simulink model "ALL_JP360_DBW_V6_5_1103"  (R2022a)
settings: Solver=FixedStepAuto  StartTime=0.0  StopTime=inf  FixedStep=0.01  RelTol=1e-3  EnableMultiTasking=on
model workspace (MAT data in the model file):
  g = 9.8
undefined symbols (not defined in the file or in its folder): canChannel, delta_v_p, IPM_Line_C0, IPM_Line_C1, IPM_Line_C2, IPM_Line_C3, M, M_p, MRR_ObjDistX, MRR_ObjDistY, MRR_ObjFusionCamID, MRR_ObjFusionSig, MRR_ObjID, MRR_ObjRelVelX, MRR_ObjRelVelY, MRR_ObjType, MRR_ObjUpdFlg, none, obj_vaild, untracktime, V, videoinput
libraries: canfdmsglib x230, canfdlib x76, slpidlib x24, simulink x18, dspstat3 x14, ctrlSharedLib x1, simulink_extras x1, imaqlib x1, realtime_pacer_lib x1, dspvision x1, visionsinks x1
(part 45 of 55)

== system ALL_JP360_DBW_V6_5_1103/MsgFromCAN/VR_ADCU_MsgFromCAN/VR_ADCU_IPM_Traffic_01_0x670 ==
  VR_ADCU_IPM_Traffic_01_0x670FromInData : Inport  OutDataTypeStr=Bus:CAN_FD_MESSAGE_BUS
  Bus Creator : BusCreator  Inputs=11  OutDataTypeStr=Bus:VR_ADCU_IPM_Traffic_01_0x670  NonVirtualBus=on
  CAN FD Unpack : canfdmsglib/CAN FD Unpack  CANdbFile=HiFire_T360_P789_1R1V_Pri_Matrix_CAN_V2.3_20220810.dbc  MsgList=(none)  MsgName=IPM_Traffic_01_0x670  ProtocolMode=CAN FD  MsgIDType=Standard (11-bit identifier)  MsgIdentifier=1648  MsgLength=20  SignalInfo={'IPM_TrafficSign01_BlockCounter','13','11','BE','unsigned','Standard','0','1','0','0','2047';'IPM_TrafficSign01_Checksum','152','16','BE','unsigned','Standard','0','1','0','0','65535';'IPM_TrafficSign01_Confidence','86','6','BE','unsigned','Standard','0','2','0','0','100';'IPM_TrafficSign01_Count','56','8','BE','unsigned','Standard','0','1','0','0','255';'IPM_TrafficSign01_ID','21','8','BE','unsigned','Standard','0','1','0','0','255';'IPM_TrafficSign01_MsgCounter','136','4','BE','unsigned','Standard','0','1','0','0','15';'IPM_TrafficSign01_PositionX','25','12','BE','unsigned','Standard','0','0.0625','0','0','254.9375';'IPM_TrafficSign01_PositionY','43','14','BE','unsigned','Standard','0','0.0078125','-64','-64','63.9922';'IPM_TrafficSign01_PositionZ','49','10','BE','unsigned','Standard','0','0.05','0','0','51.15';'IPM_TrafficSign01_Shape','76','4','BE','unsigned','Standard','0','1','0','0','15';'IPM_TrafficSign01_Type','64','8','BE','unsigned','Standard','0','1','0','0','255'}  IDPort=off  TimestampPort=off  ErrorPort=off  RemotePort=off  LengthPort=off  StatusPort=off  BRSPort=off  ESIPort=off  DLCPort=off  ApplyMinMax=off
      settings: SourceProductBaseCode=ME,XP,VN  DataFormat=CANdb specified signals
  Data Type Conversion1 : DataTypeConversion  OutDataTypeStr=int16  SaturateOnIntegerOverflow=off  RndMeth=Floor
  Data Type Conversion10 : DataTypeConversion  OutDataTypeStr=int8  SaturateOnIntegerOverflow=off  RndMeth=Floor
  Data Type Conversion11 : DataTypeConversion  OutDataTypeStr=uint8  SaturateOnIntegerOverflow=off  RndMeth=Floor
  Data Type Conversion2 : DataTypeConversion  OutDataTypeStr=uint16  SaturateOnIntegerOverflow=off  RndMeth=Floor
  Data Type Conversion3 : DataTypeConversion  OutDataTypeStr=int8  SaturateOnIntegerOverflow=off  RndMeth=Floor
  Data Type Conversion4 : DataTypeConversion  OutDataTypeStr=uint8  SaturateOnIntegerOverflow=off  RndMeth=Floor
  Data Type Conversion5 : DataTypeConversion  OutDataTypeStr=uint8  SaturateOnIntegerOverflow=off  RndMeth=Floor
  Data Type Conversion6 : DataTypeConversion  OutDataTypeStr=int8  SaturateOnIntegerOverflow=off  RndMeth=Floor
  Data Type Conversion7 : DataTypeConversion  OutDataTypeStr=single  SaturateOnIntegerOverflow=off  RndMeth=Floor
  Data Type Conversion8 : DataTypeConversion  OutDataTypeStr=single  SaturateOnIntegerOverflow=off  RndMeth=Floor
  Data Type Conversion9 : DataTypeConversion  OutDataTypeStr=single  SaturateOnIntegerOverflow=off  RndMeth=Floor
  VR_ADCU_IPM_Traffic_01_0x670FromOutData : Outport  OutDataTypeStr=Bus:VR_ADCU_IPM_Traffic_01_0x670
  wires:
  CAN FD Unpack/1 -> Data Type Conversion1/1
  CAN FD Unpack/2 -> Data Type Conversion2/1
  CAN FD Unpack/3 -> Data Type Conversion3/1
  CAN FD Unpack/4 -> Data Type Conversion4/1
  CAN FD Unpack/5 -> Data Type Conversion5/1
  CAN FD Unpack/6 -> Data Type Conversion6/1
  CAN FD Unpack/7 -> Data Type Conversion7/1
  CAN FD Unpack/8 -> Data Type Conversion8/1
  CAN FD Unpack/9 -> Data Type Conversion9/1
  CAN FD Unpack/10 -> Data Type Conversion10/1
  CAN FD Unpack/11 -> Data Type Conversion11/1
  Data Type Conversion1/1 -> Bus Creator/1  "IPM_TrafficSign01_BlockCounter"
  Data Type Conversion2/1 -> Bus Creator/2  "IPM_TrafficSign01_Checksum"
  Data Type Conversion3/1 -> Bus Creator/3  "IPM_TrafficSign01_Confidence"
  Data Type Conversion4/1 -> Bus Creator/4  "IPM_TrafficSign01_Count"
  Data Type Conversion5/1 -> Bus Creator/5  "IPM_TrafficSign01_ID"
  Data Type Conversion6/1 -> Bus Creator/6  "IPM_TrafficSign01_MsgCounter"
  Data Type Conversion7/1 -> Bus Creator/7  "IPM_TrafficSign01_PositionX"
  Data Type Conversion8/1 -> Bus Creator/8  "IPM_TrafficSign01_PositionY"
  Data Type Conversion9/1 -> Bus Creator/9  "IPM_TrafficSign01_PositionZ"
  Data Type Conversion10/1 -> Bus Creator/10  "IPM_TrafficSign01_Shape"
  Data Type Conversion11/1 -> Bus Creator/11  "IPM_TrafficSign01_Type"
  Bus Creator/1 -> VR_ADCU_IPM_Traffic_01_0x670FromOutData/1  "VR_ADCU_IPM_Traffic_01_0x670FromOutData"
  VR_ADCU_IPM_Traffic_01_0x670FromInData/1 -> CAN FD Unpack/1  "VR_ADCU_IPM_Traffic_01_0x670FromInData"

== system ALL_JP360_DBW_V6_5_1103/MsgFromCAN/VR_ADCU_MsgFromCAN/VR_ADCU_IPM_Traffic_02_0x671 ==
  VR_ADCU_IPM_Traffic_02_0x671FromInData : Inport  OutDataTypeStr=Bus:CAN_FD_MESSAGE_BUS
  Bus Creator : BusCreator  Inputs=11  OutDataTypeStr=Bus:VR_ADCU_IPM_Traffic_02_0x671  NonVirtualBus=on
  CAN FD Unpack : canfdmsglib/CAN FD Unpack  CANdbFile=HiFire_T360_P789_1R1V_Pri_Matrix_CAN_V2.3_20220810.dbc  MsgList=(none)  MsgName=IPM_Traffic_02_0x671  ProtocolMode=CAN FD  MsgIDType=Standard (11-bit identifier)  MsgIdentifier=1649  MsgLength=20  SignalInfo={'IPM_TrafficSign02_BlockCounter','13','11','BE','unsigned','Standard','0','1','0','0','2047';'IPM_TrafficSign02_Checksum','152','16','BE','unsigned','Standard','0','1','0','0','65535';'IPM_TrafficSign02_Confidence','86','6','BE','unsigned','Standard','0','2','0','0','100';'IPM_TrafficSign02_Count','56','8','BE','unsigned','Standard','0','1','0','0','255';'IPM_TrafficSign02_ID','21','8','BE','unsigned','Standard','0','1','0','0','255';'IPM_TrafficSign02_MsgCounter','136','4','BE','unsigned','Standard','0','1','0','0','15';'IPM_TrafficSign02_PositionX','25','12','BE','unsigned','Standard','0','0.0625','0','0','254.9375';'IPM_TrafficSign02_PositionY','43','14','BE','unsigned','Standard','0','0.0078125','-64','-64','63.9922';'IPM_TrafficSign02_PositionZ','49','10','BE','unsigned','Standard','0','0.05','0','0','51.15';'IPM_TrafficSign02_Shape','76','4','BE','unsigned','Standard','0','1','0','0','15';'IPM_TrafficSign02_Type','64','8','BE','unsigned','Standard','0','1','0','0','255'}  IDPort=off  TimestampPort=off  ErrorPort=off  RemotePort=off  LengthPort=off  StatusPort=off  BRSPort=off  ESIPort=off  DLCPort=off  ApplyMinMax=off
      settings: SourceProductBaseCode=ME,XP,VN  DataFormat=CANdb specified signals
  Data Type Conversion1 : DataTypeConversion  OutDataTypeStr=int16  SaturateOnIntegerOverflow=off  RndMeth=Floor
  Data Type Conversion10 : DataTypeConversion  OutDataTypeStr=int8  SaturateOnIntegerOverflow=off  RndMeth=Floor
  Data Type Conversion11 : DataTypeConversion  OutDataTypeStr=uint8  SaturateOnIntegerOverflow=off  RndMeth=Floor
  Data Type Conversion2 : DataTypeConversion  OutDataTypeStr=uint16  SaturateOnIntegerOverflow=off  RndMeth=Floor
  Data Type Conversion3 : DataTypeConversion  OutDataTypeStr=int8  SaturateOnIntegerOverflow=off  RndMeth=Floor
  Data Type Conversion4 : DataTypeConversion  OutDataTypeStr=uint8  SaturateOnIntegerOverflow=off  RndMeth=Floor
  Data Type Conversion5 : DataTypeConversion  OutDataTypeStr=uint8  SaturateOnIntegerOverflow=off  RndMeth=Floor
  Data Type Conversion6 : DataTypeConversion  OutDataTypeStr=int8  SaturateOnIntegerOverflow=off  RndMeth=Floor
  Data Type Conversion7 : DataTypeConversion  OutDataTypeStr=single  SaturateOnIntegerOverflow=off  RndMeth=Floor
  Data Type Conversion8 : DataTypeConversion  OutDataTypeStr=single  SaturateOnIntegerOverflow=off  RndMeth=Floor
  Data Type Conversion9 : DataTypeConversion  OutDataTypeStr=single  SaturateOnIntegerOverflow=off  RndMeth=Floor
  VR_ADCU_IPM_Traffic_02_0x671FromOutData : Outport  OutDataTypeStr=Bus:VR_ADCU_IPM_Traffic_02_0x671
  wires:
  CAN FD Unpack/1 -> Data Type Conversion1/1
  CAN FD Unpack/2 -> Data Type Conversion2/1
  CAN FD Unpack/3 -> Data Type Conversion3/1
  CAN FD Unpack/4 -> Data Type Conversion4/1
  CAN FD Unpack/5 -> Data Type Conversion5/1
  CAN FD Unpack/6 -> Data Type Conversion6/1
  CAN FD Unpack/7 -> Data Type Conversion7/1
  CAN FD Unpack/8 -> Data Type Conversion8/1
  CAN FD Unpack/9 -> Data Type Conversion9/1
  CAN FD Unpack/10 -> Data Type Conversion10/1
  CAN FD Unpack/11 -> Data Type Conversion11/1
  Data Type Conversion1/1 -> Bus Creator/1  "IPM_TrafficSign02_BlockCounter"
  Data Type Conversion2/1 -> Bus Creator/2  "IPM_TrafficSign02_Checksum"
  Data Type Conversion3/1 -> Bus Creator/3  "IPM_TrafficSign02_Confidence"
  Data Type Conversion4/1 -> Bus Creator/4  "IPM_TrafficSign02_Count"
  Data Type Conversion5/1 -> Bus Creator/5  "IPM_TrafficSign02_ID"
  Data Type Conversion6/1 -> Bus Creator/6  "IPM_TrafficSign02_MsgCounter"
  Data Type Conversion7/1 -> Bus Creator/7  "IPM_TrafficSign02_PositionX"
  Data Type Conversion8/1 -> Bus Creator/8  "IPM_TrafficSign02_PositionY"
  Data Type Conversion9/1 -> Bus Creator/9  "IPM_TrafficSign02_PositionZ"
  Data Type Conversion10/1 -> Bus Creator/10  "IPM_TrafficSign02_Shape"
  Data Type Conversion11/1 -> Bus Creator/11  "IPM_TrafficSign02_Type"
  Bus Creator/1 -> VR_ADCU_IPM_Traffic_02_0x671FromOutData/1  "VR_ADCU_IPM_Traffic_02_0x671FromOutData"
  VR_ADCU_IPM_Traffic_02_0x671FromInData/1 -> CAN FD Unpack/1  "VR_ADCU_IPM_Traffic_02_0x671FromInData"

== system ALL_JP360_DBW_V6_5_1103/MsgFromCAN/VR_ADCU_MsgFromCAN/VR_ADCU_IPM_Traffic_03_0x672 ==
  VR_ADCU_IPM_Traffic_03_0x672FromInData : Inport  OutDataTypeStr=Bus:CAN_FD_MESSAGE_BUS
  Bus Creator : BusCreator  Inputs=11  OutDataTypeStr=Bus:VR_ADCU_IPM_Traffic_03_0x672  NonVirtualBus=on
  CAN FD Unpack : canfdmsglib/CAN FD Unpack  CANdbFile=HiFire_T360_P789_1R1V_Pri_Matrix_CAN_V2.3_20220810.dbc  MsgList=(none)  MsgName=IPM_Traffic_03_0x672  ProtocolMode=CAN FD  MsgIDType=Standard (11-bit identifier)  MsgIdentifier=1650  MsgLength=20  SignalInfo={'IPM_TrafficSign03_BlockCounter','13','11','BE','unsigned','Standard','0','1','0','0','2047';'IPM_TrafficSign03_Checksum','152','16','BE','unsigned','Standard','0','1','0','0','65535';'IPM_TrafficSign03_Confidence','86','6','BE','unsigned','Standard','0','2','0','0','100';'IPM_TrafficSign03_Count','56','8','BE','unsigned','Standard','0','1','0','0','255';'IPM_TrafficSign03_ID','21','8','BE','unsigned','Standard','0','1','0','0','255';'IPM_TrafficSign03_MsgCounter','136','4','BE','unsigned','Standard','0','1','0','0','15';'IPM_TrafficSign03_PositionX','25','12','BE','unsigned','Standard','0','0.0625','0','0','254.9375';'IPM_TrafficSign03_PositionY','43','14','BE','unsigned','Standard','0','0.0078125','-64','-64','63.9922';'IPM_TrafficSign03_PositionZ','49','10','BE','unsigned','Standard','0','0.05','0','0','51.15';'IPM_TrafficSign03_Shape','76','4','BE','unsigned','Standard','0','1','0','0','15';'IPM_TrafficSign03_Type','64','8','BE','unsigned','Standard','0','1','0','0','255'}  IDPort=off  TimestampPort=off  ErrorPort=off  RemotePort=off  LengthPort=off  StatusPort=off  BRSPort=off  ESIPort=off  DLCPort=off  ApplyMinMax=off
      settings: SourceProductBaseCode=ME,XP,VN  DataFormat=CANdb specified signals
  Data Type Conversion1 : DataTypeConversion  OutDataTypeStr=int16  SaturateOnIntegerOverflow=off  RndMeth=Floor
  Data Type Conversion10 : DataTypeConversion  OutDataTypeStr=int8  SaturateOnIntegerOverflow=off  RndMeth=Floor
  Data Type Conversion11 : DataTypeConversion  OutDataTypeStr=uint8  SaturateOnIntegerOverflow=off  RndMeth=Floor
  Data Type Conversion2 : DataTypeConversion  OutDataTypeStr=uint16  SaturateOnIntegerOverflow=off  RndMeth=Floor
  Data Type Conversion3 : DataTypeConversion  OutDataTypeStr=int8  SaturateOnIntegerOverflow=off  RndMeth=Floor
  Data Type Conversion4 : DataTypeConversion  OutDataTypeStr=uint8  SaturateOnIntegerOverflow=off  RndMeth=Floor
  Data Type Conversion5 : DataTypeConversion  OutDataTypeStr=uint8  SaturateOnIntegerOverflow=off  RndMeth=Floor
  Data Type Conversion6 : DataTypeConversion  OutDataTypeStr=int8  SaturateOnIntegerOverflow=off  RndMeth=Floor
  Data Type Conversion7 : DataTypeConversion  OutDataTypeStr=single  SaturateOnIntegerOverflow=off  RndMeth=Floor
  Data Type Conversion8 : DataTypeConversion  OutDataTypeStr=single  SaturateOnIntegerOverflow=off  RndMeth=Floor
  Data Type Conversion9 : DataTypeConversion  OutDataTypeStr=single  SaturateOnIntegerOverflow=off  RndMeth=Floor
  VR_ADCU_IPM_Traffic_03_0x672FromOutData : Outport  OutDataTypeStr=Bus:VR_ADCU_IPM_Traffic_03_0x672
  wires:
  CAN FD Unpack/1 -> Data Type Conversion1/1
  CAN FD Unpack/2 -> Data Type Conversion2/1
  CAN FD Unpack/3 -> Data Type Conversion3/1
  CAN FD Unpack/4 -> Data Type Conversion4/1
  CAN FD Unpack/5 -> Data Type Conversion5/1
  CAN FD Unpack/6 -> Data Type Conversion6/1
  CAN FD Unpack/7 -> Data Type Conversion7/1
  CAN FD Unpack/8 -> Data Type Conversion8/1
  CAN FD Unpack/9 -> Data Type Conversion9/1
  CAN FD Unpack/10 -> Data Type Conversion10/1
  CAN FD Unpack/11 -> Data Type Conversion11/1
  Data Type Conversion1/1 -> Bus Creator/1  "IPM_TrafficSign03_BlockCounter"
  Data Type Conversion2/1 -> Bus Creator/2  "IPM_TrafficSign03_Checksum"
  Data Type Conversion3/1 -> Bus Creator/3  "IPM_TrafficSign03_Confidence"
  Data Type Conversion4/1 -> Bus Creator/4  "IPM_TrafficSign03_Count"
  Data Type Conversion5/1 -> Bus Creator/5  "IPM_TrafficSign03_ID"
  Data Type Conversion6/1 -> Bus Creator/6  "IPM_TrafficSign03_MsgCounter"
  Data Type Conversion7/1 -> Bus Creator/7  "IPM_TrafficSign03_PositionX"
  Data Type Conversion8/1 -> Bus Creator/8  "IPM_TrafficSign03_PositionY"
  Data Type Conversion9/1 -> Bus Creator/9  "IPM_TrafficSign03_PositionZ"
  Data Type Conversion10/1 -> Bus Creator/10  "IPM_TrafficSign03_Shape"
  Data Type Conversion11/1 -> Bus Creator/11  "IPM_TrafficSign03_Type"
  Bus Creator/1 -> VR_ADCU_IPM_Traffic_03_0x672FromOutData/1  "VR_ADCU_IPM_Traffic_03_0x672FromOutData"
  VR_ADCU_IPM_Traffic_03_0x672FromInData/1 -> CAN FD Unpack/1  "VR_ADCU_IPM_Traffic_03_0x672FromInData"

== system ALL_JP360_DBW_V6_5_1103/MsgFromCAN/VR_ADCU_MsgFromCAN/VR_ADCU_IPM_Traffic_04_0x673 ==
  VR_ADCU_IPM_Traffic_04_0x673FromInData : Inport  OutDataTypeStr=Bus:CAN_FD_MESSAGE_BUS
  Bus Creator : BusCreator  Inputs=11  OutDataTypeStr=Bus:VR_ADCU_IPM_Traffic_04_0x673  NonVirtualBus=on
  CAN FD Unpack : canfdmsglib/CAN FD Unpack  CANdbFile=HiFire_T360_P789_1R1V_Pri_Matrix_CAN_V2.3_20220810.dbc  MsgList=(none)  MsgName=IPM_Traffic_04_0x673  ProtocolMode=CAN FD  MsgIDType=Standard (11-bit identifier)  MsgIdentifier=1651  MsgLength=20  SignalInfo={'IPM_TrafficSign04_BlockCounter','13','11','BE','unsigned','Standard','0','1','0','0','2047';'IPM_TrafficSign04_Checksum','152','16','BE','unsigned','Standard','0','1','0','0','65535';'IPM_TrafficSign04_Confidence','86','6','BE','unsigned','Standard','0','2','0','0','100';'IPM_TrafficSign04_Count','56','8','BE','unsigned','Standard','0','1','0','0','255';'IPM_TrafficSign04_ID','21','8','BE','unsigned','Standard','0','1','0','0','255';'IPM_TrafficSign04_MsgCounter','136','4','BE','unsigned','Standard','0','1','0','0','15';'IPM_TrafficSign04_PositionX','25','12','BE','unsigned','Standard','0','0.0625','0','0','254.9375';'IPM_TrafficSign04_PositionY','43','14','BE','unsigned','Standard','0','0.0078125','-64','-64','63.9922';'IPM_TrafficSign04_PositionZ','49','10','BE','unsigned','Standard','0','0.05','0','0','51.15';'IPM_TrafficSign04_Shape','76','4','BE','unsigned','Standard','0','1','0','0','15';'IPM_TrafficSign04_Type','64','8','BE','unsigned','Standard','0','1','0','0','255'}  IDPort=off  TimestampPort=off  ErrorPort=off  RemotePort=off  LengthPort=off  StatusPort=off  BRSPort=off  ESIPort=off  DLCPort=off  ApplyMinMax=off
      settings: SourceProductBaseCode=ME,XP,VN  DataFormat=CANdb specified signals
  Data Type Conversion1 : DataTypeConversion  OutDataTypeStr=int16  SaturateOnIntegerOverflow=off  RndMeth=Floor
  Data Type Conversion10 : DataTypeConversion  OutDataTypeStr=int8  SaturateOnIntegerOverflow=off  RndMeth=Floor
  Data Type Conversion11 : DataTypeConversion  OutDataTypeStr=uint8  SaturateOnIntegerOverflow=off  RndMeth=Floor
  Data Type Conversion2 : DataTypeConversion  OutDataTypeStr=uint16  SaturateOnIntegerOverflow=off  RndMeth=Floor
  Data Type Conversion3 : DataTypeConversion  OutDataTypeStr=int8  SaturateOnIntegerOverflow=off  RndMeth=Floor
  Data Type Conversion4 : DataTypeConversion  OutDataTypeStr=uint8  SaturateOnIntegerOverflow=off  RndMeth=Floor
  Data Type Conversion5 : DataTypeConversion  OutDataTypeStr=uint8  SaturateOnIntegerOverflow=off  RndMeth=Floor
  Data Type Conversion6 : DataTypeConversion  OutDataTypeStr=int8  SaturateOnIntegerOverflow=off  RndMeth=Floor
  Data Type Conversion7 : DataTypeConversion  OutDataTypeStr=single  SaturateOnIntegerOverflow=off  RndMeth=Floor
  Data Type Conversion8 : DataTypeConversion  OutDataTypeStr=single  SaturateOnIntegerOverflow=off  RndMeth=Floor
  Data Type Conversion9 : DataTypeConversion  OutDataTypeStr=single  SaturateOnIntegerOverflow=off  RndMeth=Floor
  VR_ADCU_IPM_Traffic_04_0x673FromOutData : Outport  OutDataTypeStr=Bus:VR_ADCU_IPM_Traffic_04_0x673
  wires:
  CAN FD Unpack/1 -> Data Type Conversion1/1
  CAN FD Unpack/2 -> Data Type Conversion2/1
  CAN FD Unpack/3 -> Data Type Conversion3/1
  CAN FD Unpack/4 -> Data Type Conversion4/1
  CAN FD Unpack/5 -> Data Type Conversion5/1
  CAN FD Unpack/6 -> Data Type Conversion6/1
  CAN FD Unpack/7 -> Data Type Conversion7/1
  CAN FD Unpack/8 -> Data Type Conversion8/1
  CAN FD Unpack/9 -> Data Type Conversion9/1
  CAN FD Unpack/10 -> Data Type Conversion10/1
  CAN FD Unpack/11 -> Data Type Conversion11/1
  Data Type Conversion1/1 -> Bus Creator/1  "IPM_TrafficSign04_BlockCounter"
  Data Type Conversion2/1 -> Bus Creator/2  "IPM_TrafficSign04_Checksum"
  Data Type Conversion3/1 -> Bus Creator/3  "IPM_TrafficSign04_Confidence"
  Data Type Conversion4/1 -> Bus Creator/4  "IPM_TrafficSign04_Count"
  Data Type Conversion5/1 -> Bus Creator/5  "IPM_TrafficSign04_ID"
  Data Type Conversion6/1 -> Bus Creator/6  "IPM_TrafficSign04_MsgCounter"
  Data Type Conversion7/1 -> Bus Creator/7  "IPM_TrafficSign04_PositionX"
  Data Type Conversion8/1 -> Bus Creator/8  "IPM_TrafficSign04_PositionY"
  Data Type Conversion9/1 -> Bus Creator/9  "IPM_TrafficSign04_PositionZ"
  Data Type Conversion10/1 -> Bus Creator/10  "IPM_TrafficSign04_Shape"
  Data Type Conversion11/1 -> Bus Creator/11  "IPM_TrafficSign04_Type"
  Bus Creator/1 -> VR_ADCU_IPM_Traffic_04_0x673FromOutData/1  "VR_ADCU_IPM_Traffic_04_0x673FromOutData"
  VR_ADCU_IPM_Traffic_04_0x673FromInData/1 -> CAN FD Unpack/1  "VR_ADCU_IPM_Traffic_04_0x673FromInData"

== system ALL_JP360_DBW_V6_5_1103/MsgFromCAN/VR_ADCU_MsgFromCAN/VR_ADCU_IPM_Traffic_05_0x674 ==
  VR_ADCU_IPM_Traffic_05_0x674FromInData : Inport  OutDataTypeStr=Bus:CAN_FD_MESSAGE_BUS
  Bus Creator : BusCreator  Inputs=11  OutDataTypeStr=Bus:VR_ADCU_IPM_Traffic_05_0x674  NonVirtualBus=on
  CAN FD Unpack : canfdmsglib/CAN FD Unpack  CANdbFile=HiFire_T360_P789_1R1V_Pri_Matrix_CAN_V2.3_20220810.dbc  MsgList=(none)  MsgName=IPM_Traffic_05_0x674  ProtocolMode=CAN FD  MsgIDType=Standard (11-bit identifier)  MsgIdentifier=1652  MsgLength=20  SignalInfo={'IPM_TrafficSign05_BlockCounter','13','11','BE','unsigned','Standard','0','1','0','0','2047';'IPM_TrafficSign05_Checksum','152','16','BE','unsigned','Standard','0','1','0','0','65535';'IPM_TrafficSign05_Confidence','86','6','BE','unsigned','Standard','0','2','0','0','100';'IPM_TrafficSign05_Count','56','8','BE','unsigned','Standard','0','1','0','0','255';'IPM_TrafficSign05_ID','21','8','BE','unsigned','Standard','0','1','0','0','255';'IPM_TrafficSign05_MsgCounter','136','4','BE','unsigned','Standard','0','1','0','0','15';'IPM_TrafficSign05_PositionX','25','12','BE','unsigned','Standard','0','0.0625','0','0','254.9375';'IPM_TrafficSign05_PositionY','43','14','BE','unsigned','Standard','0','0.0078125','-64','-64','63.9922';'IPM_TrafficSign05_PositionZ','49','10','BE','unsigned','Standard','0','0.05','0','0','51.15';'IPM_TrafficSign05_Shape','76','4','BE','unsigned','Standard','0','1','0','0','15';'IPM_TrafficSign05_Type','64','8','BE','unsigned','Standard','0','1','0','0','255'}  IDPort=off  TimestampPort=off  ErrorPort=off  RemotePort=off  LengthPort=off  StatusPort=off  BRSPort=off  ESIPort=off  DLCPort=off  ApplyMinMax=off
      settings: SourceProductBaseCode=ME,XP,VN  DataFormat=CANdb specified signals
  Data Type Conversion1 : DataTypeConversion  OutDataTypeStr=int16  SaturateOnIntegerOverflow=off  RndMeth=Floor
  Data Type Conversion10 : DataTypeConversion  OutDataTypeStr=int8  SaturateOnIntegerOverflow=off  RndMeth=Floor
  Data Type Conversion11 : DataTypeConversion  OutDataTypeStr=uint8  SaturateOnIntegerOverflow=off  RndMeth=Floor
  Data Type Conversion2 : DataTypeConversion  OutDataTypeStr=uint16  SaturateOnIntegerOverflow=off  RndMeth=Floor
  Data Type Conversion3 : DataTypeConversion  OutDataTypeStr=int8  SaturateOnIntegerOverflow=off  RndMeth=Floor
  Data Type Conversion4 : DataTypeConversion  OutDataTypeStr=uint8  SaturateOnIntegerOverflow=off  RndMeth=Floor
  Data Type Conversion5 : DataTypeConversion  OutDataTypeStr=uint8  SaturateOnIntegerOverflow=off  RndMeth=Floor
  Data Type Conversion6 : DataTypeConversion  OutDataTypeStr=int8  SaturateOnIntegerOverflow=off  RndMeth=Floor
  Data Type Conversion7 : DataTypeConversion  OutDataTypeStr=single  SaturateOnIntegerOverflow=off  RndMeth=Floor
  Data Type Conversion8 : DataTypeConversion  OutDataTypeStr=single  SaturateOnIntegerOverflow=off  RndMeth=Floor
  Data Type Conversion9 : DataTypeConversion  OutDataTypeStr=single  SaturateOnIntegerOverflow=off  RndMeth=Floor
  VR_ADCU_IPM_Traffic_05_0x674FromOutData : Outport  OutDataTypeStr=Bus:VR_ADCU_IPM_Traffic_05_0x674
  wires:
  CAN FD Unpack/1 -> Data Type Conversion1/1
  CAN FD Unpack/2 -> Data Type Conversion2/1
  CAN FD Unpack/3 -> Data Type Conversion3/1
  CAN FD Unpack/4 -> Data Type Conversion4/1
  CAN FD Unpack/5 -> Data Type Conversion5/1
  CAN FD Unpack/6 -> Data Type Conversion6/1
  CAN FD Unpack/7 -> Data Type Conversion7/1
  CAN FD Unpack/8 -> Data Type Conversion8/1
  CAN FD Unpack/9 -> Data Type Conversion9/1
  CAN FD Unpack/10 -> Data Type Conversion10/1
  CAN FD Unpack/11 -> Data Type Conversion11/1
  Data Type Conversion1/1 -> Bus Creator/1  "IPM_TrafficSign05_BlockCounter"
  Data Type Conversion2/1 -> Bus Creator/2  "IPM_TrafficSign05_Checksum"
  Data Type Conversion3/1 -> Bus Creator/3  "IPM_TrafficSign05_Confidence"
  Data Type Conversion4/1 -> Bus Creator/4  "IPM_TrafficSign05_Count"
  Data Type Conversion5/1 -> Bus Creator/5  "IPM_TrafficSign05_ID"
  Data Type Conversion6/1 -> Bus Creator/6  "IPM_TrafficSign05_MsgCounter"
  Data Type Conversion7/1 -> Bus Creator/7  "IPM_TrafficSign05_PositionX"
  Data Type Conversion8/1 -> Bus Creator/8  "IPM_TrafficSign05_PositionY"
  Data Type Conversion9/1 -> Bus Creator/9  "IPM_TrafficSign05_PositionZ"
  Data Type Conversion10/1 -> Bus Creator/10  "IPM_TrafficSign05_Shape"
  Data Type Conversion11/1 -> Bus Creator/11  "IPM_TrafficSign05_Type"
  Bus Creator/1 -> VR_ADCU_IPM_Traffic_05_0x674FromOutData/1  "VR_ADCU_IPM_Traffic_05_0x674FromOutData"
  VR_ADCU_IPM_Traffic_05_0x674FromInData/1 -> CAN FD Unpack/1  "VR_ADCU_IPM_Traffic_05_0x674FromInData"

== system ALL_JP360_DBW_V6_5_1103/MsgFromCAN/VR_ADCU_MsgFromCAN/VR_ADCU_IPM_Traffic_06_0x675 ==
  VR_ADCU_IPM_Traffic_06_0x675FromInData : Inport  OutDataTypeStr=Bus:CAN_FD_MESSAGE_BUS
  Bus Creator : BusCreator  Inputs=11  OutDataTypeStr=Bus:VR_ADCU_IPM_Traffic_06_0x675  NonVirtualBus=on
  CAN FD Unpack : canfdmsglib/CAN FD Unpack  CANdbFile=HiFire_T360_P789_1R1V_Pri_Matrix_CAN_V2.3_20220810.dbc  MsgList=(none)  MsgName=IPM_Traffic_06_0x675  ProtocolMode=CAN FD  MsgIDType=Standard (11-bit identifier)  MsgIdentifier=1653  MsgLength=20  SignalInfo={'IPM_TrafficSign06_BlockCounter','13','11','BE','unsigned','Standard','0','1','0','0','2047';'IPM_TrafficSign06_Checksum','152','16','BE','unsigned','Standard','0','1','0','0','65535';'IPM_TrafficSign06_Confidence','86','6','BE','unsigned','Standard','0','2','0','0','100';'IPM_TrafficSign06_Count','56','8','BE','unsigned','Standard','0','1','0','0','255';'IPM_TrafficSign06_ID','21','8','BE','unsigned','Standard','0','1','0','0','255';'IPM_TrafficSign06_MsgCounter','136','4','BE','unsigned','Standard','0','1','0','0','15';'IPM_TrafficSign06_PositionX','25','12','BE','unsigned','Standard','0','0.0625','0','0','254.9375';'IPM_TrafficSign06_PositionY','43','14','BE','unsigned','Standard','0','0.0078125','-64','-64','63.9922';'IPM_TrafficSign06_PositionZ','49','10','BE','unsigned','Standard','0','0.05','0','0','51.15';'IPM_TrafficSign06_Shape','76','4','BE','unsigned','Standard','0','1','0','0','15';'IPM_TrafficSign06_Type','64','8','BE','unsigned','Standard','0','1','0','0','255'}  IDPort=off  TimestampPort=off  ErrorPort=off  RemotePort=off  LengthPort=off  StatusPort=off  BRSPort=off  ESIPort=off  DLCPort=off  ApplyMinMax=off
      settings: SourceProductBaseCode=ME,XP,VN  DataFormat=CANdb specified signals
  Data Type Conversion1 : DataTypeConversion  OutDataTypeStr=int16  SaturateOnIntegerOverflow=off  RndMeth=Floor
  Data Type Conversion10 : DataTypeConversion  OutDataTypeStr=int8  SaturateOnIntegerOverflow=off  RndMeth=Floor
  Data Type Conversion11 : DataTypeConversion  OutDataTypeStr=uint8  SaturateOnIntegerOverflow=off  RndMeth=Floor
  Data Type Conversion2 : DataTypeConversion  OutDataTypeStr=uint16  SaturateOnIntegerOverflow=off  RndMeth=Floor
  Data Type Conversion3 : DataTypeConversion  OutDataTypeStr=int8  SaturateOnIntegerOverflow=off  RndMeth=Floor
  Data Type Conversion4 : DataTypeConversion  OutDataTypeStr=uint8  SaturateOnIntegerOverflow=off  RndMeth=Floor
  Data Type Conversion5 : DataTypeConversion  OutDataTypeStr=uint8  SaturateOnIntegerOverflow=off  RndMeth=Floor
  Data Type Conversion6 : DataTypeConversion  OutDataTypeStr=int8  SaturateOnIntegerOverflow=off  RndMeth=Floor
  Data Type Conversion7 : DataTypeConversion  OutDataTypeStr=single  SaturateOnIntegerOverflow=off  RndMeth=Floor
  Data Type Conversion8 : DataTypeConversion  OutDataTypeStr=single  SaturateOnIntegerOverflow=off  RndMeth=Floor
  Data Type Conversion9 : DataTypeConversion  OutDataTypeStr=single  SaturateOnIntegerOverflow=off  RndMeth=Floor
  VR_ADCU_IPM_Traffic_06_0x675FromOutData : Outport  OutDataTypeStr=Bus:VR_ADCU_IPM_Traffic_06_0x675
  wires:
  CAN FD Unpack/1 -> Data Type Conversion1/1
  CAN FD Unpack/2 -> Data Type Conversion2/1
  CAN FD Unpack/3 -> Data Type Conversion3/1
  CAN FD Unpack/4 -> Data Type Conversion4/1
  CAN FD Unpack/5 -> Data Type Conversion5/1
  CAN FD Unpack/6 -> Data Type Conversion6/1
  CAN FD Unpack/7 -> Data Type Conversion7/1
  CAN FD Unpack/8 -> Data Type Conversion8/1
  CAN FD Unpack/9 -> Data Type Conversion9/1
  CAN FD Unpack/10 -> Data Type Conversion10/1
  CAN FD Unpack/11 -> Data Type Conversion11/1
  Data Type Conversion1/1 -> Bus Creator/1  "IPM_TrafficSign06_BlockCounter"
  Data Type Conversion2/1 -> Bus Creator/2  "IPM_TrafficSign06_Checksum"
  Data Type Conversion3/1 -> Bus Creator/3  "IPM_TrafficSign06_Confidence"
  Data Type Conversion4/1 -> Bus Creator/4  "IPM_TrafficSign06_Count"
  Data Type Conversion5/1 -> Bus Creator/5  "IPM_TrafficSign06_ID"
  Data Type Conversion6/1 -> Bus Creator/6  "IPM_TrafficSign06_MsgCounter"
  Data Type Conversion7/1 -> Bus Creator/7  "IPM_TrafficSign06_PositionX"
  Data Type Conversion8/1 -> Bus Creator/8  "IPM_TrafficSign06_PositionY"
  Data Type Conversion9/1 -> Bus Creator/9  "IPM_TrafficSign06_PositionZ"
  Data Type Conversion10/1 -> Bus Creator/10  "IPM_TrafficSign06_Shape"
  Data Type Conversion11/1 -> Bus Creator/11  "IPM_TrafficSign06_Type"
  Bus Creator/1 -> VR_ADCU_IPM_Traffic_06_0x675FromOutData/1  "VR_ADCU_IPM_Traffic_06_0x675FromOutData"
  VR_ADCU_IPM_Traffic_06_0x675FromInData/1 -> CAN FD Unpack/1  "VR_ADCU_IPM_Traffic_06_0x675FromInData"

== system ALL_JP360_DBW_V6_5_1103/MsgFromCAN/VR_ADCU_MsgFromCAN/VR_ADCU_IPM_VLC_0x393 ==
  VR_ADCU_IPM_VLC_0x393FromInData : Inport  OutDataTypeStr=Bus:CAN_FD_MESSAGE_BUS
  Bus Creator : BusCreator  Inputs=4  OutDataTypeStr=Bus:VR_ADCU_IPM_VLC_0x393  NonVirtualBus=on
  CAN FD Unpack : canfdmsglib/CAN FD Unpack  CANdbFile=HiFire_T360_P789_1R1V_Pri_Matrix_CAN_V2.3_20220810.dbc  MsgList=(none)  MsgName=IPM_VLC_0x393  ProtocolMode=CAN FD  MsgIDType=Standard (11-bit identifier)  MsgIdentifier=915  MsgLength=8  SignalInfo={'ACC_Torque_Request','16','16','BE','unsigned','Standard','0','0.5','-15000','-15000','15000';'ACC_Torque_Request_Status','7','1','BE','unsigned','Standard','0','1','0','0','1';'Checksum_0x293','56','8','BE','unsigned','Standard','0','1','0','0','255';'RollingCounter_0x293','48','4','BE','unsigned','Standard','0','1','0','0','15'}  IDPort=off  TimestampPort=off  ErrorPort=off  RemotePort=off  LengthPort=off  StatusPort=off  BRSPort=off  ESIPort=off  DLCPort=off  ApplyMinMax=off
      settings: SourceProductBaseCode=ME,XP,VN  DataFormat=CANdb specified signals
  Data Type Conversion1 : DataTypeConversion  OutDataTypeStr=single  SaturateOnIntegerOverflow=off  RndMeth=Floor
  Data Type Conversion2 : DataTypeConversion  OutDataTypeStr=boolean  SaturateOnIntegerOverflow=off  RndMeth=Floor
  Data Type Conversion3 : DataTypeConversion  OutDataTypeStr=uint8  SaturateOnIntegerOverflow=off  RndMeth=Floor
  Data Type Conversion4 : DataTypeConversion  OutDataTypeStr=int8  SaturateOnIntegerOverflow=off  RndMeth=Floor
  VR_ADCU_IPM_VLC_0x393FromOutData : Outport  OutDataTypeStr=Bus:VR_ADCU_IPM_VLC_0x393
  wires:
  CAN FD Unpack/1 -> Data Type Conversion1/1
  CAN FD Unpack/2 -> Data Type Conversion2/1
  CAN FD Unpack/3 -> Data Type Conversion3/1
  CAN FD Unpack/4 -> Data Type Conversion4/1
  Data Type Conversion1/1 -> Bus Creator/1  "ACC_Torque_Request"
  Data Type Conversion2/1 -> Bus Creator/2  "ACC_Torque_Request_Status"
  Data Type Conversion3/1 -> Bus Creator/3  "Checksum_0x293"
  Data Type Conversion4/1 -> Bus Creator/4  "RollingCounter_0x293"
  Bus Creator/1 -> VR_ADCU_IPM_VLC_0x393FromOutData/1  "VR_ADCU_IPM_VLC_0x393FromOutData"
  VR_ADCU_IPM_VLC_0x393FromInData/1 -> CAN FD Unpack/1  "VR_ADCU_IPM_VLC_0x393FromInData"

== system ALL_JP360_DBW_V6_5_1103/MsgFromCAN/VR_ADCU_MsgFromCAN/VR_ADCU_MRR_0x338 ==
  VR_ADCU_MRR_0x338FromInData : Inport  OutDataTypeStr=Bus:CAN_FD_MESSAGE_BUS
  Bus Creator : BusCreator  Inputs=7  OutDataTypeStr=Bus:VR_ADCU_MRR_0x338  NonVirtualBus=on
  CAN FD Unpack : canfdmsglib/CAN FD Unpack  CANdbFile=HiFire_T360_P789_1R1V_Pri_Matrix_CAN_V2.3_20220810.dbc  MsgList=(none)  MsgName=MRR_0x338  ProtocolMode=CAN FD  MsgIDType=Standard (11-bit identifier)  MsgIdentifier=824  MsgLength=8  SignalInfo={'ACC_TgtAx','53','11','BE','unsigned','Standard','0','0.05','-5','-5','7.75';'ACC_TgtAxLowerComftBand','8','8','BE','unsigned','Standard','0','0.05','0','0','3.2';'ACC_TgtAxLowerLim','24','8','BE','unsigned','Standard','0','0.1','-12.7','-12.7','0';'ACC_TgtAxUpperComftBand','0','8','BE','unsigned','Standard','0','0.05','0','0','3.2';'ACC_TgtAxUpperLim','16','8','BE','unsigned','Standard','0','0.1','0','0','12.7';'Checksum_0x238','56','8','BE','unsigned','Standard','0','1','0','0','255';'RollingCounter_0x238','48','4','BE','unsigned','Standard','0','1','0','0','15'}  IDPort=off  TimestampPort=off  ErrorPort=off  RemotePort=off  LengthPort=off  StatusPort=off  BRSPort=off  ESIPort=off  DLCPort=off  ApplyMinMax=off
      settings: SourceProductBaseCode=ME,XP,VN  DataFormat=CANdb specified signals
  Data Type Conversion{1..5} (5 alike) : DataTypeConversion  OutDataTypeStr=single  SaturateOnIntegerOverflow=off  RndMeth=Floor
  Data Type Conversion6 : DataTypeConversion  OutDataTypeStr=uint8  SaturateOnIntegerOverflow=off  RndMeth=Floor
  Data Type Conversion7 : DataTypeConversion  OutDataTypeStr=int8  SaturateOnIntegerOverflow=off  RndMeth=Floor
  VR_ADCU_MRR_0x338FromOutData : Outport  OutDataTypeStr=Bus:VR_ADCU_MRR_0x338
  wires:
  CAN FD Unpack/1 -> Data Type Conversion1/1
  CAN FD Unpack/2 -> Data Type Conversion2/1
  CAN FD Unpack/3 -> Data Type Conversion3/1
  CAN FD Unpack/4 -> Data Type Conversion4/1
  CAN FD Unpack/5 -> Data Type Conversion5/1
  CAN FD Unpack/6 -> Data Type Conversion6/1
  CAN FD Unpack/7 -> Data Type Conversion7/1
  Data Type Conversion1/1 -> Bus Creator/1  "ACC_TgtAx"
  Data Type Conversion2/1 -> Bus Creator/2  "ACC_TgtAxLowerComftBand"
  Data Type Conversion3/1 -> Bus Creator/3  "ACC_TgtAxLowerLim"
  Data Type Conversion4/1 -> Bus Creator/4  "ACC_TgtAxUpperComftBand"
  Data Type Conversion5/1 -> Bus Creator/5  "ACC_TgtAxUpperLim"
  Data Type Conversion6/1 -> Bus Creator/6  "Checksum_0x238"
  Data Type Conversion7/1 -> Bus Creator/7  "RollingCounter_0x238"
  Bus Creator/1 -> VR_ADCU_MRR_0x338FromOutData/1  "VR_ADCU_MRR_0x338FromOutData"
  VR_ADCU_MRR_0x338FromInData/1 -> CAN FD Unpack/1  "VR_ADCU_MRR_0x338FromInData"

== system ALL_JP360_DBW_V6_5_1103/MsgFromCAN/VR_ADCU_MsgFromCAN/VR_ADCU_MRR_0x339 ==
  VR_ADCU_MRR_0x339FromInData : Inport  OutDataTypeStr=Bus:CAN_FD_MESSAGE_BUS
  Bus Creator : BusCreator  Inputs=16  OutDataTypeStr=Bus:VR_ADCU_MRR_0x339  NonVirtualBus=on
  CAN FD Unpack : canfdmsglib/CAN FD Unpack  CANdbFile=HiFire_T360_P789_1R1V_Pri_Matrix_CAN_V2.3_20220810.dbc  MsgList=(none)  MsgName=MRR_0x339  ProtocolMode=CAN FD  MsgIDType=Standard (11-bit identifier)  MsgIdentifier=825  MsgLength=8  SignalInfo={'ABA_Level','8','2','BE','unsigned','Standard','0','1','0','0','3';'ABA_Req','23','1','BE','unsigned','Standard','0','1','0','0','1';'ABP_Req','21','1','BE','unsigned','Standard','0','1','0','0','1';'ACC_BrakePreferred','1','1','BE','unsigned','Standard','0','1','0','0','1';'ACC_DriveOff','15','1','BE','unsigned','Standard','0','1','0','0','1';'ACC_StandstillReq','14','1','BE','unsigned','Standard','0','1','0','0','1';'ACC_Status','3','3','BE','unsigned','Standard','0','1','0','0','7';'ACC_VLCMinBrakingReq','0','1','BE','unsigned','Standard','0','1','0','0','1';'ACC_VLCShutdownMode','6','2','BE','unsigned','Standard','0','1','0','0','3';'AEB_Req','13','1','BE','unsigned','Standard','0','1','0','0','1';'AEB_TgtAx','32','16','BE','unsigned','Standard','0','0.05','-16','-16','16';'AWB_Level','16','4','BE','unsigned','Standard','0','1','0','0','15';'AWB_Req','22','1','BE','unsigned','Standard','0','1','0','0','1';'Checksum_0x239','56','8','BE','unsigned','Standard','0','1','0','0','255';'EBA_Req','12','1','BE','unsigned','Standard','0','1','0','0','1';'RollingCounter_0x239','48','4','BE','unsigned','Standard','0','1','0','0','15'}  IDPort=off  TimestampPort=off  ErrorPort=off  RemotePort=off  LengthPort=off  StatusPort=off  BRSPort=off  ESIPort=off  DLCPort=off  ApplyMinMax=off
      settings: SourceProductBaseCode=ME,XP,VN  DataFormat=CANdb specified signals
  Data Type Conversion{1,7,9,12,16} (5 alike) : DataTypeConversion  OutDataTypeStr=int8  SaturateOnIntegerOverflow=off  RndMeth=Floor
  Data Type Conversion{2..6,8,10,13,15} (9 alike) : DataTypeConversion  OutDataTypeStr=boolean  SaturateOnIntegerOverflow=off  RndMeth=Floor
  Data Type Conversion11 : DataTypeConversion  OutDataTypeStr=single  SaturateOnIntegerOverflow=off  RndMeth=Floor
  Data Type Conversion14 : DataTypeConversion  OutDataTypeStr=uint8  SaturateOnIntegerOverflow=off  RndMeth=Floor
  VR_ADCU_MRR_0x339FromOutData : Outport  OutDataTypeStr=Bus:VR_ADCU_MRR_0x339
  wires:
  CAN FD Unpack/1 -> Data Type Conversion1/1
  CAN FD Unpack/2 -> Data Type Conversion2/1
  CAN FD Unpack/3 -> Data Type Conversion3/1
  CAN FD Unpack/4 -> Data Type Conversion4/1
  CAN FD Unpack/5 -> Data Type Conversion5/1
  CAN FD Unpack/6 -> Data Type Conversion6/1
  CAN FD Unpack/7 -> Data Type Conversion7/1
  CAN FD Unpack/8 -> Data Type Conversion8/1
  CAN FD Unpack/9 -> Data Type Conversion9/1
  CAN FD Unpack/10 -> Data Type Conversion10/1
  CAN FD Unpack/11 -> Data Type Conversion11/1
  CAN FD Unpack/12 -> Data Type Conversion12/1
  CAN FD Unpack/13 -> Data Type Conversion13/1
  CAN FD Unpack/14 -> Data Type Conversion14/1
  CAN FD Unpack/15 -> Data Type Conversion15/1
  CAN FD Unpack/16 -> Data Type Conversion16/1
  Data Type Conversion1/1 -> Bus Creator/1  "ABA_Level"
  Data Type Conversion2/1 -> Bus Creator/2  "ABA_Req"
  Data Type Conversion3/1 -> Bus Creator/3  "ABP_Req"
  Data Type Conversion4/1 -> Bus Creator/4  "ACC_BrakePreferred"
  Data Type Conversion5/1 -> Bus Creator/5  "ACC_DriveOff"
  Data Type Conversion6/1 -> Bus Creator/6  "ACC_StandstillReq"
  Data Type Conversion7/1 -> Bus Creator/7  "ACC_Status"
  Data Type Conversion8/1 -> Bus Creator/8  "ACC_VLCMinBrakingReq"
  Data Type Conversion9/1 -> Bus Creator/9  "ACC_VLCShutdownMode"
  Data Type Conversion10/1 -> Bus Creator/10  "AEB_Req"
  Data Type Conversion11/1 -> Bus Creator/11  "AEB_TgtAx"
  Data Type Conversion12/1 -> Bus Creator/12  "AWB_Level"
  Data Type Conversion13/1 -> Bus Creator/13  "AWB_Req"
  Data Type Conversion14/1 -> Bus Creator/14  "Checksum_0x239"
  Data Type Conversion15/1 -> Bus Creator/15  "EBA_Req"
  Data Type Conversion16/1 -> Bus Creator/16  "RollingCounter_0x239"
  Bus Creator/1 -> VR_ADCU_MRR_0x339FromOutData/1  "VR_ADCU_MRR_0x339FromOutData"
  VR_ADCU_MRR_0x339FromInData/1 -> CAN FD Unpack/1  "VR_ADCU_MRR_0x339FromInData"

== system ALL_JP360_DBW_V6_5_1103/MsgFromCAN/VR_ADCU_MsgFromCAN/VR_ADCU_MRR_0x346 ==
  VR_ADCU_MRR_0x346FromInData : Inport  OutDataTypeStr=Bus:CAN_FD_MESSAGE_BUS
  Bus Creator : BusCreator  Inputs=19  OutDataTypeStr=Bus:VR_ADCU_MRR_0x346  NonVirtualBus=on
  CAN FD Unpack : canfdmsglib/CAN FD Unpack  CANdbFile=HiFire_T360_P789_1R1V_Pri_Matrix_CAN_V2.3_20220810.dbc  MsgList=(none)  MsgName=MRR_0x346  ProtocolMode=CAN FD  MsgIDType=Standard (11-bit identifier)  MsgIdentifier=838  MsgLength=8  SignalInfo={'ACC_EngineStartstop','28','2','BE','unsigned','Standard','0','1','0','0','3';'ACC_FailInfo','19','1','BE','unsigned','Standard','0','1','0','0','1';'ACC_ModeHMI','16','3','BE','unsigned','Standard','0','1','0','0','7';'ACC_ObjDetected','8','1','BE','unsigned','Standard','0','1','0','0','1';'ACC_SpdSetValue','15','9','BE','unsigned','Standard','0','0.5','0','0','255.5';'ACC_TakeOverReq','20','1','BE','unsigned','Standard','0','1','0','0','1';'ACC_TarObjBarDis','12','3','BE','unsigned','Standard','0','1','0','0','7';'ACC_Textinfo','52','6','BE','unsigned','Standard','0','1','0','0','63';'ACC_TimeGapSet','9','3','BE','unsigned','Standard','0','1','0','0','7';'AEB_Status','25','3','BE','unsigned','Standard','0','1','0','0','7';'Checksum_0x246','56','8','BE','unsigned','Standard','0','1','0','0','255';'FCW_PedWarningLevel1','21','1','BE','unsigned','Standard','0','1','0','0','1';'FCW_PedWarningLevel2','24','1','BE','unsigned','Standard','0','1','0','0','1';'FCW_Sensitive','22','2','BE','unsigned','Standard','0','1','0','0','3';'FCW_Status','37','3','BE','unsigned','Standard','0','1','0','0','7';'FCW_WarningLevel1','31','1','BE','unsigned','Standard','0','1','0','0','1';'FCW_WarningLevel2','30','1','BE','unsigned','Standard','0','1','0','0','1';'Obj_Speed','42','8','BE','unsigned','Standard','0','1','0','0','255';'RollingCounter_0x246','48','4','BE','unsigned','Standard','0','1','0','0','15'}  IDPort=off  TimestampPort=off  ErrorPort=off  RemotePort=off  LengthPort=off  StatusPort=off  BRSPort=off  ESIPort=off  DLCPort=off  ApplyMinMax=off
      settings: SourceProductBaseCode=ME,XP,VN  DataFormat=CANdb specified signals
  Data Type Conversion{1,3,7..10,14..15,19} (9 alike) : DataTypeConversion  OutDataTypeStr=int8  SaturateOnIntegerOverflow=off  RndMeth=Floor
  Data Type Conversion11 : DataTypeConversion  OutDataTypeStr=uint8  SaturateOnIntegerOverflow=off  RndMeth=Floor
  Data Type Conversion{2,4,6,12..13,16..17} (7 alike) : DataTypeConversion  OutDataTypeStr=boolean  SaturateOnIntegerOverflow=off  RndMeth=Floor
  Data Type Conversion18 : DataTypeConversion  OutDataTypeStr=uint8  SaturateOnIntegerOverflow=off  RndMeth=Floor
  Data Type Conversion5 : DataTypeConversion  OutDataTypeStr=single  SaturateOnIntegerOverflow=off  RndMeth=Floor
  VR_ADCU_MRR_0x346FromOutData : Outport  OutDataTypeStr=Bus:VR_ADCU_MRR_0x346
  wires:
  CAN FD Unpack/1 -> Data Type Conversion1/1
  CAN FD Unpack/2 -> Data Type Conversion2/1
  CAN FD Unpack/3 -> Data Type Conversion3/1
  CAN FD Unpack/4 -> Data Type Conversion4/1
  CAN FD Unpack/5 -> Data Type Conversion5/1
  CAN FD Unpack/6 -> Data Type Conversion6/1
  CAN FD Unpack/7 -> Data Type Conversion7/1
  CAN FD Unpack/8 -> Data Type Conversion8/1
  CAN FD Unpack/9 -> Data Type Conversion9/1
  CAN FD Unpack/10 -> Data Type Conversion10/1
  CAN FD Unpack/11 -> Data Type Conversion11/1
  CAN FD Unpack/12 -> Data Type Conversion12/1
  CAN FD Unpack/13 -> Data Type Conversion13/1
  CAN FD Unpack/14 -> Data Type Conversion14/1
  CAN FD Unpack/15 -> Data Type Conversion15/1
  CAN FD Unpack/16 -> Data Type Conversion16/1
  CAN FD Unpack/17 -> Data Type Conversion17/1
  CAN FD Unpack/18 -> Data Type Conversion18/1
  CAN FD Unpack/19 -> Data Type Conversion19/1
  Data Type Conversion1/1 -> Bus Creator/1  "ACC_EngineStartstop"
  Data Type Conversion2/1 -> Bus Creator/2  "ACC_FailInfo"
  Data Type Conversion3/1 -> Bus Creator/3  "ACC_ModeHMI"
  Data Type Conversion4/1 -> Bus Creator/4  "ACC_ObjDetected"
  Data Type Conversion5/1 -> Bus Creator/5  "ACC_SpdSetValue"
  Data Type Conversion6/1 -> Bus Creator/6  "ACC_TakeOverReq"
  Data Type Conversion7/1 -> Bus Creator/7  "ACC_TarObjBarDis"
  Data Type Conversion8/1 -> Bus Creator/8  "ACC_Textinfo"
  Data Type Conversion9/1 -> Bus Creator/9  "ACC_TimeGapSet"
  Data Type Conversion10/1 -> Bus Creator/10  "AEB_Status"
  Data Type Conversion11/1 -> Bus Creator/11  "Checksum_0x246"
  Data Type Conversion12/1 -> Bus Creator/12  "FCW_PedWarningLevel1"
  Data Type Conversion13/1 -> Bus Creator/13  "FCW_PedWarningLevel2"
  Data Type Conversion14/1 -> Bus Creator/14  "FCW_Sensitive"
  Data Type Conversion15/1 -> Bus Creator/15  "FCW_Status"
  Data Type Conversion16/1 -> Bus Creator/16  "FCW_WarningLevel1"
  Data Type Conversion17/1 -> Bus Creator/17  "FCW_WarningLevel2"
  Data Type Conversion18/1 -> Bus Creator/18  "Obj_Speed"
  Data Type Conversion19/1 -> Bus Creator/19  "RollingCounter_0x246"
  Bus Creator/1 -> VR_ADCU_MRR_0x346FromOutData/1  "VR_ADCU_MRR_0x346FromOutData"
  VR_ADCU_MRR_0x346FromInData/1 -> CAN FD Unpack/1  "VR_ADCU_MRR_0x346FromInData"

== system ALL_JP360_DBW_V6_5_1103/MsgFromCAN/VR_ADCU_MsgFromCAN/VR_ADCU_MRR_FRObj_0x379 ==
  VR_ADCU_MRR_FRObj_0x379FromInData : Inport  OutDataTypeStr=Bus:CAN_FD_MESSAGE_BUS
  Bus Creator : BusCreator  Inputs=8  OutDataTypeStr=Bus:VR_ADCU_MRR_FRObj_0x379  NonVirtualBus=on
  CAN FD Unpack : canfdmsglib/CAN FD Unpack  CANdbFile=HiFire_T360_P789_1R1V_Pri_Matrix_CAN_V2.3_20220810.dbc  MsgList=(none)  MsgName=MRR_FRObj_0x379  ProtocolMode=CAN FD  MsgIDType=Standard (11-bit identifier)  MsgIdentifier=889  MsgLength=8  SignalInfo={'MRR_FFTargetDetection','54','1','BE','unsigned','Standard','0','1','0','0','1';'MRR_FF_Obj_0x_class','40','3','BE','unsigned','Standard','0','1','0','0','7';'MRR_FF_Object_dx','36','12','BE','unsigned','Standard','0','0.0625','0','0','255.875';'MRR_FF_Object_dy','43','9','BE','unsigned','Standard','0','0.0625','-15','-15','15';'MRR_F_Obj_0x_class','16','3','BE','unsigned','Standard','0','1','0','0','7';'MRR_F_Object_dx','12','12','BE','unsigned','Standard','0','0.0625','0','0','255.875';'MRR_F_Object_dy','19','9','BE','unsigned','Standard','0','0.0625','-15','-15','15';'MRR_PedDetection','55','1','BE','unsigned','Standard','0','1','0','0','1'}  IDPort=off  TimestampPort=off  ErrorPort=off  RemotePort=off  LengthPort=off  StatusPort=off  BRSPort=off  ESIPort=off  DLCPort=off  ApplyMinMax=off
      settings: SourceProductBaseCode=ME,XP,VN  DataFormat=CANdb specified signals
  Data Type Conversion1 : DataTypeConversion  OutDataTypeStr=boolean  SaturateOnIntegerOverflow=off  RndMeth=Floor
  Data Type Conversion2 : DataTypeConversion  OutDataTypeStr=int8  SaturateOnIntegerOverflow=off  RndMeth=Floor
  Data Type Conversion{3..4,6..7} (4 alike) : DataTypeConversion  OutDataTypeStr=single  SaturateOnIntegerOverflow=off  RndMeth=Floor
  Data Type Conversion5 : DataTypeConversion  OutDataTypeStr=int8  SaturateOnIntegerOverflow=off  RndMeth=Floor
  Data Type Conversion8 : DataTypeConversion  OutDataTypeStr=boolean  SaturateOnIntegerOverflow=off  RndMeth=Floor
  VR_ADCU_MRR_FRObj_0x379FromOutData : Outport  OutDataTypeStr=Bus:VR_ADCU_MRR_FRObj_0x379
  wires:
  CAN FD Unpack/1 -> Data Type Conversion1/1
  CAN FD Unpack/2 -> Data Type Conversion2/1
  CAN FD Unpack/3 -> Data Type Conversion3/1
  CAN FD Unpack/4 -> Data Type Conversion4/1
  CAN FD Unpack/5 -> Data Type Conversion5/1
  CAN FD Unpack/6 -> Data Type Conversion6/1
  CAN FD Unpack/7 -> Data Type Conversion7/1
  CAN FD Unpack/8 -> Data Type Conversion8/1
  Data Type Conversion1/1 -> Bus Creator/1  "MRR_FFTargetDetection"
  Data Type Conversion2/1 -> Bus Creator/2  "MRR_FF_Obj_0x_class"
  Data Type Conversion3/1 -> Bus Creator/3  "MRR_FF_Object_dx"
  Data Type Conversion4/1 -> Bus Creator/4  "MRR_FF_Object_dy"
  Data Type Conversion5/1 -> Bus Creator/5  "MRR_F_Obj_0x_class"
  Data Type Conversion6/1 -> Bus Creator/6  "MRR_F_Object_dx"
  Data Type Conversion7/1 -> Bus Creator/7  "MRR_F_Object_dy"
  Data Type Conversion8/1 -> Bus Creator/8  "MRR_PedDetection"
  Bus Creator/1 -> VR_ADCU_MRR_FRObj_0x379FromOutData/1  "VR_ADCU_MRR_FRObj_0x379FromOutData"
  VR_ADCU_MRR_FRObj_0x379FromInData/1 -> CAN FD Unpack/1  "VR_ADCU_MRR_FRObj_0x379FromInData"

== system ALL_JP360_DBW_V6_5_1103/MsgFromCAN/VR_ADCU_MsgFromCAN/VR_ADCU_MRR_LRObj_0x580 ==
  VR_ADCU_MRR_LRObj_0x580FromInData : Inport  OutDataTypeStr=Bus:CAN_FD_MESSAGE_BUS
  Bus Creator : BusCreator  Inputs=8  OutDataTypeStr=Bus:VR_ADCU_MRR_LRObj_0x580  NonVirtualBus=on
  CAN FD Unpack : canfdmsglib/CAN FD Unpack  CANdbFile=HiFire_T360_P789_1R1V_Pri_Matrix_CAN_V2.3_20220810.dbc  MsgList=(none)  MsgName=MRR_LRObj_0x580  ProtocolMode=CAN FD  MsgIDType=Standard (11-bit identifier)  MsgIdentifier=1408  MsgLength=8  SignalInfo={'MRR_L_Obj_0x_class','16','3','BE','unsigned','Standard','0','1','0','0','7';'MRR_L_Object_dx','12','12','BE','unsigned','Standard','0','0.0625','0','0','255.875';'MRR_L_Object_dy','19','9','BE','unsigned','Standard','0','0.0625','-15','-15','15';'MRR_LeftTargetDetection','54','1','BE','unsigned','Standard','0','1','0','0','1';'MRR_R_Obj_0x_class','40','3','BE','unsigned','Standard','0','1','0','0','7';'MRR_R_Object_dx','36','12','BE','unsigned','Standard','0','0.0625','0','0','255.875';'MRR_R_Object_dy','43','9','BE','unsigned','Standard','0','0.0625','-15','-15','15';'MRR_RightTargetDetection','55','1','BE','unsigned','Standard','0','1','0','0','1'}  IDPort=off  TimestampPort=off  ErrorPort=off  RemotePort=off  LengthPort=off  StatusPort=off  BRSPort=off  ESIPort=off  DLCPort=off  ApplyMinMax=off
      settings: SourceProductBaseCode=ME,XP,VN  DataFormat=CANdb specified signals
  Data Type Conversion1 : DataTypeConversion  OutDataTypeStr=int8  SaturateOnIntegerOverflow=off  RndMeth=Floor
  Data Type Conversion{2..3,6..7} (4 alike) : DataTypeConversion  OutDataTypeStr=single  SaturateOnIntegerOverflow=off  RndMeth=Floor
  Data Type Conversion4 : DataTypeConversion  OutDataTypeStr=boolean  SaturateOnIntegerOverflow=off  RndMeth=Floor
  Data Type Conversion5 : DataTypeConversion  OutDataTypeStr=int8  SaturateOnIntegerOverflow=off  RndMeth=Floor
  Data Type Conversion8 : DataTypeConversion  OutDataTypeStr=boolean  SaturateOnIntegerOverflow=off  RndMeth=Floor
  VR_ADCU_MRR_LRObj_0x580FromOutData : Outport  OutDataTypeStr=Bus:VR_ADCU_MRR_LRObj_0x580
  wires:
  CAN FD Unpack/1 -> Data Type Conversion1/1
  CAN FD Unpack/2 -> Data Type Conversion2/1
  CAN FD Unpack/3 -> Data Type Conversion3/1
  CAN FD Unpack/4 -> Data Type Conversion4/1
  CAN FD Unpack/5 -> Data Type Conversion5/1
  CAN FD Unpack/6 -> Data Type Conversion6/1
  CAN FD Unpack/7 -> Data Type Conversion7/1
  CAN FD Unpack/8 -> Data Type Conversion8/1
  Data Type Conversion1/1 -> Bus Creator/1  "MRR_L_Obj_0x_class"
  Data Type Conversion2/1 -> Bus Creator/2  "MRR_L_Object_dx"
  Data Type Conversion3/1 -> Bus Creator/3  "MRR_L_Object_dy"
  Data Type Conversion4/1 -> Bus Creator/4  "MRR_LeftTargetDetection"
  Data Type Conversion5/1 -> Bus Creator/5  "MRR_R_Obj_0x_class"
  Data Type Conversion6/1 -> Bus Creator/6  "MRR_R_Object_dx"
  Data Type Conversion7/1 -> Bus Creator/7  "MRR_R_Object_dy"
  Data Type Conversion8/1 -> Bus Creator/8  "MRR_RightTargetDetection"
  Bus Creator/1 -> VR_ADCU_MRR_LRObj_0x580FromOutData/1  "VR_ADCU_MRR_LRObj_0x580FromOutData"
  VR_ADCU_MRR_LRObj_0x580FromInData/1 -> CAN FD Unpack/1  "VR_ADCU_MRR_LRObj_0x580FromInData"
